simulink subsystem "MPC7_nlpsol"  (R2022b)
settings: Solver=VariableStepAuto  StartTime=0.0  StopTime=10.0  RelTol=1e-3
undefined symbols (not defined in the file): param_MPC7, param_weight_init
settings Model: Creator=emu  LastModifiedBy=rslstudent
settings OptimizationCC: ReuseModelBlockBuffer=on

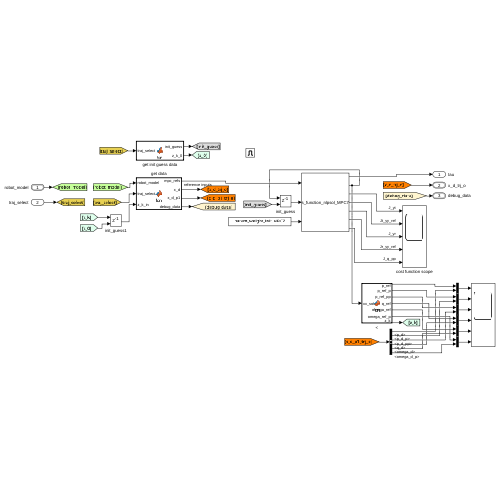
[thumbnail: Simulink's stored preview of the top-level diagram]
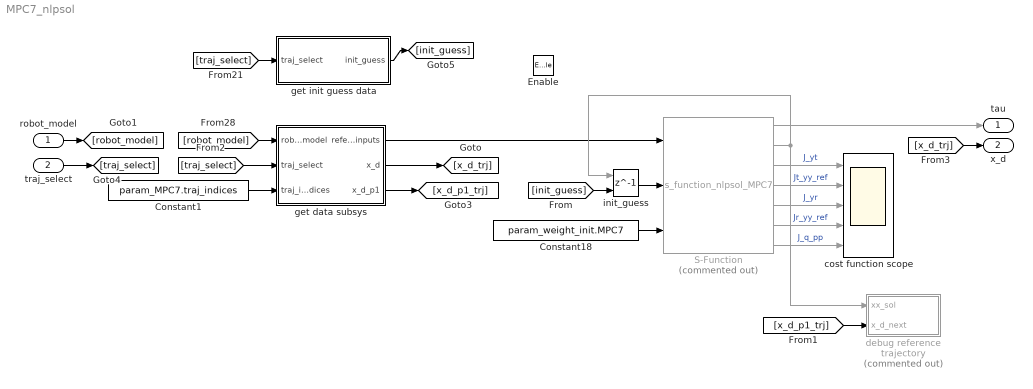
== system MPC7_nlpsol ==
  robot_model : Inport  OutDataTypeStr=Bus: robot_model
  traj_select : Inport  Port=2
  Enable : EnablePort
  Constant1 : Constant  Value=param_MPC7.traj_indices
  Constant18 : Constant  Value=param_weight_init.MPC7  VectorParams1D=off
  S-Function : S-Function  Commented=on  FunctionName=s_function_nlpsol_MPC7  Parameters='s_functions/fr3_no_hand_6dof/MPC7.casadi', 'MPC7'  SFunctionModules='MPC7'  SFunctionDeploymentMode=off  EnableBusSupport=off
  cost function scope : Scope  NumInputPorts=5
  debug reference trajectory : Subsystem  Commented=on
  get data subsys : Subsystem
  get init guess data : MATLAB Function  TreatAsAtomicUnit=on
  init_guess : Delay  DelayLength=1  InitialConditionSource=Input port  InitialCondition=1
      settings: InputPortMap=u0,p4
  tau : Outport
  x_d : Outport  Port=2  OutDataTypeStr=Bus: x_d
  wires:
  get data subsys/3(x_d_p1) -> [x_d_p1_trj]
  get data subsys/2(x_d) -> [x_d_trj]
  get data subsys/1(reference inputs) -> S-Function/1
  Constant1/1 -> get data subsys/3(traj_indices)
  [traj_select] -> get data subsys/2(traj_select)
  [robot_model] -> get data subsys/1(robot_model)
  [x_d_trj] -> x_d/1
  [x_d_p1_trj] -> debug reference trajectory/2(x_d_next)
  S-Function/5 -> cost function scope/3  "J_yr"
  S-Function/7 -> cost function scope/5  "J_q_pp"
  Constant18/1 -> S-Function/3
  S-Function/4 -> cost function scope/2  "Jt_yy_ref"
  S-Function/2 -> init_guess/1, debug reference trajectory/1(xx_sol)
  get init guess data/1(init_guess) -> [init_guess]
  init_guess/1 -> S-Function/2
  traj_select/1 -> [traj_select]
  [init_guess] -> init_guess/2
  S-Function/1 -> tau/1
  robot_model/1 -> [robot_model]
  S-Function/6 -> cost function scope/4  "Jr_yy_ref"
  S-Function/3 -> cost function scope/1  "J_yt"
  [traj_select] -> get init guess data/1(traj_select)

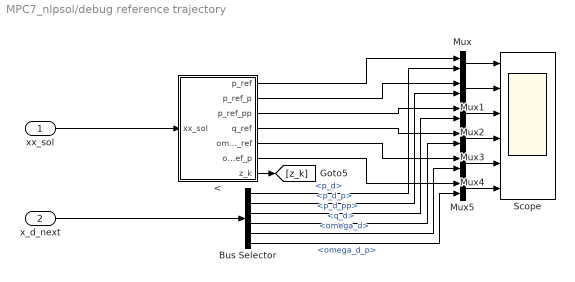
== system MPC7_nlpsol/debug reference trajectory ==
  xx_sol : Inport
  x_d_next : Inport  Port=2  OutDataTypeStr=Bus: x_d
  < : MATLAB Function  TreatAsAtomicUnit=on
  Bus Selector : BusSelector  OutputSignals=p_d,p_d_p,p_d_pp,q_d,omega_d,omega_d_p
  Mux{,1..5} (6 alike) : Mux  Inputs=2
  Scope : Scope  NumInputPorts=6
  wires:
  Mux4/1 -> Scope/5
  Bus Selector/3 -> Mux2/2  "<p_d_pp>"
  </5(omega_ref) -> Mux4/1
  xx_sol/1 -> </1(xx_sol)
  Bus Selector/5 -> Mux4/2  "<omega_d>"
  </1(p_ref) -> Mux/1
  </7(z_k) -> [z_k]
  </2(p_ref_p) -> Mux1/1
  Bus Selector/4 -> Mux3/2  "<q_d>"
  </6(omega_ref_p) -> Mux5/1
  Mux/1 -> Scope/1
  x_d_next/1 -> Bus Selector/1
  Bus Selector/2 -> Mux1/2  "<p_d_p>"
  </4(q_ref) -> Mux3/1
  Bus Selector/6 -> Mux5/2  "<omega_d_p>"
  Mux2/1 -> Scope/3
  Mux3/1 -> Scope/4
  Bus Selector/1 -> Mux/2  "<p_d>"
  Mux5/1 -> Scope/6
  </3(p_ref_pp) -> Mux2/1
  Mux1/1 -> Scope/2

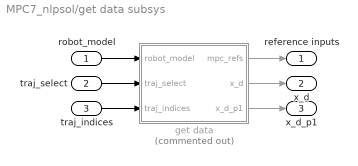
== system MPC7_nlpsol/get data subsys ==
  robot_model : Inport  OutDataTypeStr=Bus: robot_model
  traj_select : Inport  Port=2
  traj_indices : Inport  Port=3
  get data : MATLAB Function  Commented=on  TreatAsAtomicUnit=on
  reference inputs : Outport
  x_d : Outport  Port=2  OutDataTypeStr=Bus: x_d
  x_d_p1 : Outport  Port=3  OutDataTypeStr=Bus: x_d
  wires:
  robot_model/1 -> get data/1(robot_model)
  traj_indices/1 -> get data/3(traj_indices)
  get data/3(x_d_p1) -> x_d_p1/1
  get data/1(mpc_refs) -> reference inputs/1
  get data/2(x_d) -> x_d/1
  traj_select/1 -> get data/2(traj_select)

== matlab function MPC7_nlpsol/debug reference trajectory/< ==
  data: xx_sol input; p_ref output; param_MPC7 parameter; p_ref_p output; p_ref_pp output; q_ref output; omega_ref output; omega_ref_p output; z_k output
function [p_ref, p_ref_p, p_ref_pp, q_ref, omega_ref, omega_ref_p, z_k] = fcn(xx_sol, param_MPC7)

if ~isscalar(xx_sol)
    param_MPC = param_MPC7;
    
    pp_indices = param_MPC.pp;
    pp_dim = param_MPC.pp_dim;
    
    rr_indices = param_MPC.rr;
    rr_dim = param_MPC.rr_dim;
    
    qq_indices = param_MPC.qq;
    qq_dim = param_MPC.qq_dim;
    
    pp = reshape(xx_sol(pp_indices), pp_dim);
    rr = reshape(xx_sol(rr_indices), rr_dim);
    qq = reshape(xx_sol(qq_indices), qq_dim);
    
    p_ref = pp(1:3, 1 + (1));
    p_ref_p = pp(4:6, 1 + (1));
    p_ref_pp = pp(7:9, 1 + (1));
    
    q_ref = rr(1:4, 1 + (1));
    omega_ref = rr(5:7, 1 + (1));
    omega_ref_p = rr(8:10, 1 + (1));
    
    z_k = [p_ref; p_ref_p; q_ref; omega_ref];
else
    p_ref = zeros(3,1);
    p_ref_p = zeros(3,1);
    p_ref_pp = zeros(3,1);
    
    q_ref = zeros(4,1);
    omega_ref = zeros(3,1);
    omega_ref_p = zeros(3,1);
    
    z_k = [p_ref; p_ref_p; q_ref; omega_ref];
end

== matlab function MPC7_nlpsol/get data subsys/get data ==
  settings: updateMethod=DISCRETE  sampleTime=param_global.Ta
  data: mpc_refs output; robot_model input Bus: robot_model; x_d output Bus: x_d; param_traj_data parameter; traj_select input; x_d_p1 output Bus: x_d; traj_indices input
function [mpc_refs, x_d, x_d_p1] = fcn(robot_model, param_traj_data, traj_select, traj_indices)
persistent cnt;

if(isempty(cnt))
    cnt = 1;
end

traj_indices = traj_indices + (cnt-1);

% Parameters
q    = robot_model.q;      % generalized coordinates
q_p  = robot_model.q_p;  % time derivative of generalized coordinates

x_k = [q;q_p];

% Assemble vector of recieved output measurements
p_d     = param_traj_data.p_d(   1:3, traj_indices, traj_select);
p_d_p     = param_traj_data.p_d_p(   1:3, traj_indices, traj_select);
p_d_pp     = param_traj_data.p_d_pp(   1:3, traj_indices, traj_select);

% RPY XYZ angles
Phi_d = param_traj_data.Phi_d(      1:3, traj_indices, traj_select ); % (Phi_0 ... Phi_N)
Phi_d_p = param_traj_data.Phi_d_p(  1:3, traj_indices, traj_select ); % (Phi_p_0 ... Phi_p_N)
Phi_d_pp = param_traj_data.Phi_d_pp(1:3, traj_indices, traj_select ); % (Phi_pp_0 ... Phi_pp_N)

q_d    = param_traj_data.q_d(       1:4, traj_indices, traj_select);
%q_d_p  = param_traj_data.q_d_p(     1:4, traj_indices, traj_select);
%q_d_pp = param_traj_data.q_d_pp(    1:4, traj_indices, traj_select);

omega_d   = param_traj_data.omega_d(  1:3, traj_indices, traj_select);
omega_d_p = param_traj_data.omega_d_p(1:3, traj_indices, traj_select);

alpha_d    = param_traj_data.alpha_d(           :, traj_indices, traj_select);
alpha_d_p  = param_traj_data.alpha_d_p(         :, traj_indices, traj_select);
alpha_d_pp = param_traj_data.alpha_d_pp(        :, traj_indices, traj_select);
rot_ax_d   = param_traj_data.rot_ax_d(          :, traj_indices, traj_select);
alpha_d_offset = param_traj_data.alpha_d_offset(:, traj_indices, traj_select);
q_d_rel = param_traj_data.q_d_rel(              :, traj_indices, traj_select);

y_d = [p_d; Phi_d];
y_d_p = [p_d_p; Phi_d_p];
y_d_pp = [p_d_pp; Phi_d_pp];
z_k = [y_d(1:3,1); y_d_p(1:3,1); y_d(4:6,1); y_d_p(4:6,1);]; %EULER!!

%% Reference out
mpc_refs = [x_k(:); z_k(:); y_d(:); y_d_p(:); y_d_pp(:)];

%% TRAJECTORY OUT
x_d.p_d       = param_traj_data.p_d(1:3, cnt , traj_select);    %y0
x_d.p_d_p     = param_traj_data.p_d_p(1:3, cnt , traj_select);  %y0p
x_d.p_d_pp    = param_traj_data.p_d_pp(1:3, cnt , traj_select); %y0pp
x_d.Phi_d     = param_traj_data.Phi_d(:, cnt , traj_select);
x_d.Phi_d_p   = param_traj_data.Phi_d_p(:, cnt, traj_select);
x_d.Phi_d_pp  = param_traj_data.Phi_d_pp(:,cnt, traj_select);
x_d.R_d       = param_traj_data.R_d(:,:, cnt, traj_select);
x_d.q_d       = q_d(1:4, 1);
x_d.q_d_p     = param_traj_data.q_d_p(1:4, cnt, traj_select);
x_d.q_d_pp    = param_traj_data.q_d_pp(1:4, cnt, traj_select);
x_d.omega_d   = omega_d(1:3, 1);
x_d.omega_d_p = omega_d_p(1:3, 1);
x_d.alpha_d    = alpha_d(:, 1);
x_d.alpha_d_p  = alpha_d_p(:, 1);
x_d.alpha_d_pp = alpha_d_pp(:, 1);
x_d.rot_ax_d   = rot_ax_d(:, 1);
x_d.alpha_d_offset = alpha_d_offset(:, 1);
x_d.q_d_rel = q_d_rel(:, 1);

%% NEXT REFERENCE TRAJECTORY OUT
x_d_p1.p_d       = param_traj_data.p_d(1:3, cnt+1 , traj_select);    %y0
x_d_p1.p_d_p     = param_traj_data.p_d_p(1:3, cnt+1 , traj_select);  %y0p
x_d_p1.p_d_pp    = param_traj_data.p_d_pp(1:3, cnt+1 , traj_select); %y0pp
x_d_p1.Phi_d     = param_traj_data.Phi_d(:, cnt+1 , traj_select);
x_d_p1.Phi_d_p   = param_traj_data.Phi_d_p(:, cnt+1, traj_select);
x_d_p1.Phi_d_pp  = param_traj_data.Phi_d_pp(:,cnt+1, traj_select);
x_d_p1.R_d       = param_traj_data.R_d(:,:, cnt+1, traj_select);
x_d_p1.q_d       = q_d(1:4, 2);
x_d_p1.q_d_p     = param_traj_data.q_d_p(1:4, cnt+1, traj_select);
x_d_p1.q_d_pp    = param_traj_data.q_d_pp(1:4, cnt+1, traj_select);
x_d_p1.omega_d   = omega_d(1:3, 2);
x_d_p1.omega_d_p = omega_d_p(1:3, 2);
x_d_p1.alpha_d    = alpha_d(:, 2);
x_d_p1.alpha_d_p  = alpha_d_p(:, 2);
x_d_p1.alpha_d_pp = alpha_d_pp(:, 2);
x_d_p1.rot_ax_d   = rot_ax_d(:, 2);
x_d_p1.alpha_d_offset = alpha_d_offset(:, 2);
x_d_p1.q_d_rel = q_d_rel(:, 2);

cnt = cnt+1;

== matlab function MPC7_nlpsol/get init guess data ==
  data: traj_select input; param_MPC7_init_guess parameter; init_guess output
function init_guess  = fcn(traj_select, param_MPC7_init_guess)

init_guess = param_MPC7_init_guess.init_guess(traj_select,:);
